simulink model "03_ee_c"  (R2023a)
settings: Solver=VariableStepDiscrete  StartTime=0.0  StopTime=6  RelTol=1e-4
PreLoadFcn:
  | Ts=10e-6;
  | fnom=50;
undefined symbols (not defined in the file): D1, D11, Delta, DiscIntNeverNeededParam, find_system
libraries: powerlib_extras x18, simulink_extras x7, spsThreePhaseVIMeasurementLib x6, spsThreePhaseTransformerTwoWindingsLib x2, spsUniversalBridgeLib x2, spsThreePhaseProgrammableVoltageSourceLib x1, spsThreePhaseMutualInductanceZ1Z0Lib x1, spsThreePhasePISectionLineLib x1, spsGroundLib x1, spsSeriesRLCBranchLib x1, spsThreePhaseSeriesRLCBranchLib x1, spsThreePhaseSeriesRLCLoadLib x1
(part 1 of 3)
Description:
  | Copyright 2008-2009 The MathWorks(TM), Inc.
settings Model: SimulationMode=accelerator  Creator=ch0272  LastModifiedBy=eagle
settings SolverCC: AlgebraicLoopSolver=TrustRegion  SolverResetMethod=Robust
settings DataIOCC: LimitDataPoints=on  SaveFinalState=on  SaveFormat=StructureWithTime  SignalLoggingSaveFormat=ModelDataLogs  ReturnWorkspaceOutputs=off
settings OptimizationCC: ExpressionDepthLimit=2147483647  InitFltsAndDblsToZero=on  LifeSpan=inf
settings DebuggingCC: UnderspecifiedInitializationDetection=Classic  MergeDetectMultiDrivingBlocksExec=none  SolverPrmCheckMsg=warning  FcnCallInpInsideContextMsg=warning  StateNameClashWarn=warning  SFUnexpectedBacktrackingDiag=warning  SFNoUnconditionalDefaultTransitionDiag=warning  SFExecutionAtInitializationDiag=none  ArithmeticOperatorsInVariantConditions=warning
settings HardwareCC: ProdBitPerPointer=32  ProdBitPerSizeT=32  ProdBitPerPtrDiffT=32  ProdLargestAtomicFloat=None  ProdIntDivRoundTo=Undefined  ProdEndianess=Unspecified  ProdWordSize=32  ProdHWDeviceType=32-bit Generic
settings ModelReferenceCC: PropagateSignalLabelsOutOfModel=off
settings SFSimCC: SimUseLocalCustomCode=off  CustomCodeUndefinedFunction=UseInterfaceOnly
settings RTWCC: RTWUseLocalCustomCode=off
settings CodeAppCC: StateflowObjectComments=on
settings GRTTargetCC: TargetLangStandard=C89/C90 (ANSI)  CombineOutputUpdateFcns=off  GRTInterface=on
settings ConfigComp: CovMetricSettings=dw  CovSaveCumulativeToWorkspaceVar=on  CovSaveSingleToWorkspaceVar=on  CovExternalEMLEnable=off  CovSFcnEnable=off
settings SimscapeCC: SimscapeNormalizeSystem=off

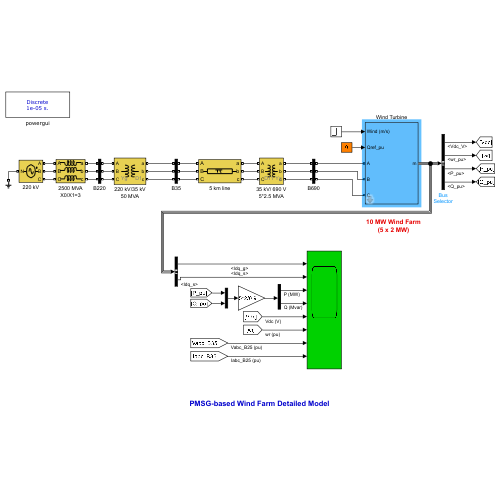
[thumbnail: Simulink's stored preview of the top-level diagram]
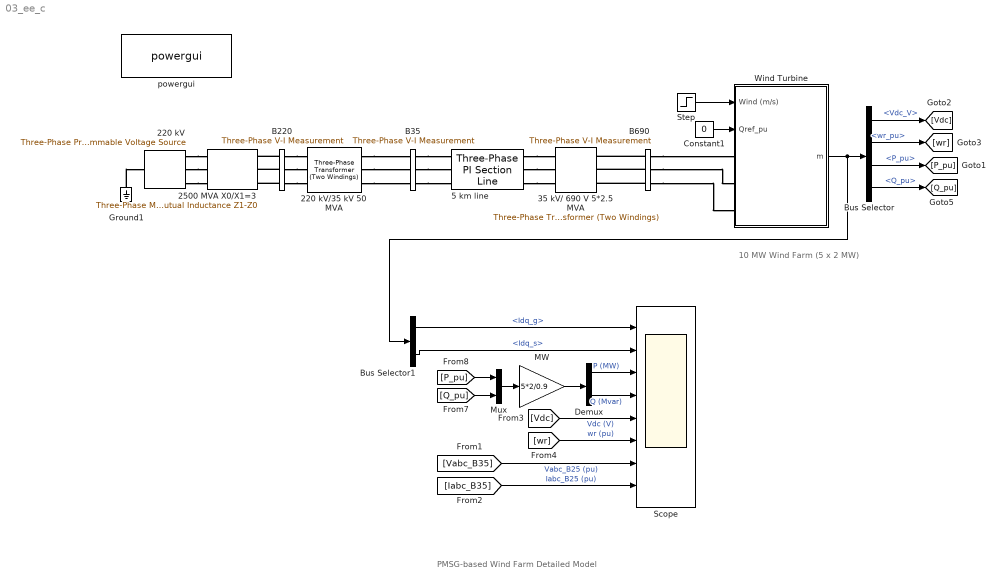
== system 03_ee_c ==
  note: 10 MW Wind Farm
      | (5 x 2 MW)
  note: PMSG-based Wind Farm Detailed Model
  220 kV : spsThreePhaseProgrammableVoltageSourceLib/Three-Phase Programmable Voltage Source  PositiveSequence=[220e3 0 fnom]  VariationEntity=Amplitude  VariationType=Table of time-amplitude pairs  VariationTypeAlt=Step  VariationStep=-0.2  VariationRate=10  VariationMagnitude=0.3  VariationFrequency=2  VariationTiming=[0.05 0.05+5/60]  VariationPhaseA=off  Amplitudes=[1 0.4 1.0]  TimeValues=[0 4 4.625]  HarmonicGeneration=off  HarmonicA=[1 -0.1 0 2]  HarmonicB=[2 0.15 35 2]*0  Timing="[0.1  2]"  BusType=swing  Pref=0  Qref=0  Qmin=-inf  Qmax=inf
  220 kV/35 kV 50 MVA : spsThreePhaseTransformerTwoWindingsLib/Three-Phase Transformer (Two Windings)  Winding1Connection=Yg  Winding2Connection=Delta (D1)  CoreType=Three single-phase transformers  SetSaturation=off  Hysteresis=off  DataFile='basic_model'  SetInitialFlux=off  Measurements=None  UNITS=pu  NominalPower=[50e6 fnom ]  Winding1="[ 220e3  0.08/30   0.05 ]"  Winding2="[ 35e3  0.08/30  0.05]"  Rm=500  Lm=500  L0=0.5  Saturation="[ 0,0  ;  0.005,1.2  ;  1.0,1.4 ]"  InitialFluxes=[ 0.8 , -0.8 , 0.7 ]  BreakLoop=off  DiscreteSolver=Trapezoidal iterative  DataType=off  TransfoNumber=0
  2500 MVA X0/X1=3 : spsThreePhaseMutualInductanceZ1Z0Lib/Three-Phase Mutual Inductance Z1-Z0  LConnTagsString=a|b|c  RConnTagsString=A|B|C  PositiveSequence="[0.1  1.0/(2*pi*fnom)] *220e3^2/2500e6"  ZeroSequence="[0.3  3.0/(2*pi*fnom)] *220e3^2/2500e6"
      settings: AttributesFormatString=\n
      settings: LibrarySourceBlock=|
      | sps_lib/Power Grid Elements/Three-Phase
      | Mutual Inductance
      | Z1-Z0
  35 kV/ 690 V 5*2.5 MVA : spsThreePhaseTransformerTwoWindingsLib/Three-Phase Transformer (Two Windings)  Winding1Connection=Delta (D11)  Winding2Connection=Yg  CoreType=Three single-phase transformers  SetSaturation=off  Hysteresis=off  DataFile='hysteresis'  SetInitialFlux=off  Measurements=None  UNITS=pu  NominalPower="[2.5e6*5  fnom]"  Winding1=[35e3 , 0.025/30 , 0.025]  Winding2=[ 690, 0.025/30 , 0.025]  Rm=500  Lm=inf  L0=0.5  Saturation=[ 0,0 ; 0.0024,1.2 ; 1.0,1.52 ]  InitialFluxes=[ 0.8 , -0.8 , 0.7 ]  BreakLoop=off  DiscreteSolver=Trapezoidal iterative  DataType=off  TransfoNumber=0
  5 km line : spsThreePhasePISectionLineLib/Three-Phase PI Section Line  LConnTagsString=a|b|c  RConnTagsString=A|B|C  Length=5  Frequency=50  Resistances=[0.1153 0.413]  Inductances=[1.05e-3 3.32e-3]  Capacitances=[11.33e-009 5.01e-009]
  B220 : spsThreePhaseVIMeasurementLib/Three-Phase V-I Measurement  VoltageMeasurement=no  SetLabelV=off  LabelV=Vabc_B120  Vpu=off  VpuLL=off  CurrentMeasurement=no  SetLabelI=on  LabelI=Iabc_B120  Ipu=off  Pbase=100e6  Vbase=120e3  OutputType=Complex  PhasorSimulation=off  PSBequivalent=0
  B35 : spsThreePhaseVIMeasurementLib/Three-Phase V-I Measurement  VoltageMeasurement=phase-to-ground  SetLabelV=on  LabelV=Vabc_B35  Vpu=on  VpuLL=off  CurrentMeasurement=yes  SetLabelI=on  LabelI=Iabc_B35  Ipu=on  Pbase=10e6  Vbase=35e3  OutputType=Complex  PhasorSimulation=off  PSBequivalent=0
  B690 : spsThreePhaseVIMeasurementLib/Three-Phase V-I Measurement  VoltageMeasurement=phase-to-ground  SetLabelV=on  LabelV=Vabc_B690  Vpu=on  VpuLL=off  CurrentMeasurement=yes  SetLabelI=on  LabelI=Iabc_B690  Ipu=on  Pbase=5*2e6  Vbase=690  OutputType=Complex  PhasorSimulation=off  PSBequivalent=0
  Bus Selector : BusSelector  OutputSignals=Vdc_V,Stator dq Frame.wr_pu,PQ&V.P_pu,PQ&V.Q_pu
  Bus Selector1 : BusSelector  OutputSignals=Grid dq Frame.Idq_g,Stator dq Frame.Idq_s
  Constant1 : Constant  Value=0
  Demux : Demux  Outputs=2
  Ground1 : spsGroundLib/Ground  LConnTagsString=a
  MW : Gain  Gain=5*2/0.9  SaturateOnIntegerOverflow=on  OutDataTypeStr=Inherit: Same as input  ParamDataTypeStr=Inherit: Same as input
  Mux : Mux  Inputs=2
  Scope : Scope  NumInputPorts=8
  Step : Step  Time=3  Before=11  After=11  SampleTime=0
  Wind Turbine : Subsystem  AncestorBlock=|  LoadFcn=%find_system(gcs,'FollowLinks', 'on', 'LookUnderMasks', 'all');  mask(Wind Turbine: Model 7){Nb_wt=5, ShowParameters=Turbine data for 1 wind turbine, nom=[2e6/0.9 690 fnom], Reactances=[ 0.0014 0.0014 ], Rs=0.0066, Flux=8.5, mec=[5e4 0 38], Vnom=690, Imax_grid_conv=1.1, RL_grid=[ 0.15 0.15/50], C_var_filter1=150e3, Vdc_nom=1200, C_DClink1=50000e-6, L_R_Boost=[0.0012     5e-3], Pmec1=2e6, wind_speed_CpMax=11, wind0=11, DisplayTurbChar=off, H_WT=4.32, Ksh=0.3, D_mutual=1.5, w_wt0=1, torque0=1, Kdc=[1.1   27.5], Ki_var_reg=0.05, Ki_volt_reg=2, Kgrid_side_cur_reg=[2  50], Kspeed=[5 20], K_PMSG_cur_reg=[2 50], Kp_pitch=15, Kcompensation=[1.5  6], pitch_max=27, pitch_rate=10, Ts=Ts}
      | DRlib/Wind Generation/Wind Turbine
      | Induction Generator
      | (Phasor Type)
      mask prompts: Nb_wt "Number of wind turbines:"; ShowParameters "Display:"; nom "Nom. power, L-L volt. and freq.: [Pn (VA), Vn (Vrms), fn (Hz)]"; Reactances "Reactances [Ld Lq] (p.u.):"; Rs "Resistance Rs :"; Flux "Flux linkage estableished by magnets"; mec "Inertia constant, friction factor, and pairs of poles: [ J  F  p ]"; Vnom "Grid-side converter nominal AC voltage (V):"; Imax_grid_conv "Grid-side converter maximum AC current (pu based on generator power and converter nominal AC voltage):"; RL_grid "Grid-side coupling inductor [ L(pu) R(pu),pu based on generator power and converter nominal AC voltage] :"; C_var_filter1 "Line filter capacitor (Q=50) (var):"; Vdc_nom "Nominal DC bus voltage (V)"; C_DClink1 "DC bus capacitor (F):"; L_R_Boost "Boost converter inductance [L(H) R(ohm)]:"; Pmec1 "Nominal mechanical output power (W):"; wind_speed_CpMax "Wind speed at nominal speed and at Cp max (must be between 6 m/s and 30 m/s) (m/s):"; wind0 "Initial wind speed (m/s):"; DisplayTurbChar "Display wind turbine power characteristics:"; H_WT "Wind turbine inertia constant H (s):"; Ksh "Shaft spring constant refer to high-speed shaft (pu of nominal mechanical torque/rad):"; D_mutual "Shaft mutual damping (pu of nominal mechanical torque/pu dw):"; w_wt0 "Turbine initial speed (pu of nominal speed):"; torque0 "Initial output torque (pu of nominal mechanical torque):"; Kdc "DC bus voltage regulator gains [Kp Ki]:"; Ki_var_reg "Grid-side converter var regulator gain [ Ki]:"; Ki_volt_reg "Grid-side converter voltage regulator gain [ Ki]:"; Kgrid_side_cur_reg "Grid-side converter current regulator gains [Kp Ki]:"; Kspeed "Speed regulator gains [Kp Ki]:"; K_PMSG_cur_reg "Stator-side converter current regulator gains [Kp Ki]:"; Kp_pitch "Pitch controller gain [Kp]:"; Kcompensation "Pitch compensation gains [Kp Ki]:"; pitch_max "Maximum pitch angle (deg):"; pitch_rate "Maximum rate of change of pitch angle (deg/s)"; Ts "Sample time (s):"
      mask help: This block implements a model of a variable speed pitch controlled wind turbine using a synchronous generator.
      mask init:
      | %Generator data
      | Pnom=nom(1)*Nb_wt;
      | Vnom_gen=nom(2);
      | Fnom=nom(3);
      | Ld=Reactances(1)/Nb_wt;
      | Lq=Reactances(2)/Nb_wt;
      | Resistance=Rs/Nb_wt;
      | J=mec(1)*Nb_wt;
      | F=mec(2);
      | p=mec(3);
      | 
      | % Converters data
      | L_RL=RL_grid(1);
      | R_RL=RL_grid(2);
      | L_Boost=L_R_Boost(1)/Nb_wt;
      | R_Boost=L_R_Boost(2)/Nb_wt;
      | Q_filter=50;
      | C_DClink=C_DClink1*Nb_wt;
      | C_var_filter=C_var_filter1*Nb_wt;
      | 
      | % Controller data
      | Freq_filter=10000;   %Hz
      | Zeta_filter=0.707;
      | Kp_dc=Kdc(1);
      | Ki_dc=Kdc(2);
      | Kp_grid_side_cur_reg=Kgrid_side_cur_reg(1);
      | Ki_grid_side_cur_reg=Kgrid_side_cur_reg(2);
      | Kp_speed=Kspeed(1);
      | Ki_speed=Kspeed(2);
      | Kp_PMSG_side_cur_reg=K_PMSG_cur_reg(1);
      | Ki_PMSG_side_cur_reg=K_PMSG_cur_reg(2);
      | Kp_compensation=Kcompensation(1);
      | Ki_compensation=Kcompensation(2);
      | Mod_index_max=1.1;
      | T_speed=5;      %Speed reference time constant (s)
      | Iq_ref_limit_time_constant=0.3; %(s)
      | Current_reg_output_limit=1.1;   %(pu)
      | Var_reg_output_hi_limit=1.1;    %(pu)
      | Var_reg_output_low_limit=0.9;   %(pu)
      | Pitch_time_constant=0.01;       %(s)
      | Freq_PWM=3000; %Hz, Inverter
      | Ts_snub=50e-6;  %Sample time to compute snubber resistance
      | 
      | 
      | % Turbine data
      | Pmec=Pmec1*Nb_wt;
      | c1 = 0.6450;
      | c2 = 116;
      | c3 = .4;
      | c4 = 5;
      | c5 = 21;
      | c6 = .00912;  % Set Pmin in stall condition (does not vary with wind_speed_Pmax)
      | c7 = .08;
      | c8 = .035;
      | theta=0;
      | CpMax=.5;
      | lambda_CpMax=9.9495;
      | 
      | c1_c8=[c1 c2 c3 c4 c5 c6 c7 c8];
      |   
      | 
      | %   Cp = c1*(c6*lambda + (-c4 - c3*(2.5 + theta) + c2*(1/(lambda + ...
      | %   c7*(2.5 + theta)) - c8/(1 + (2.5 + theta)^3)))/exp(c5*(1/(lambda + ...
      | %   c7*(2.5 + theta)) - c8/(1 + (2.5 + theta)^3))))
      | 
      | 
      |         %%%%%%%%%%%%%%%%%%%%%%%%%%%%%%%%%%%%%%%%%%%%%%%%%%%%%%%%%%%%%%%%%%%%%%%%%%%
      |         % Operation at Cp max
      |         %%%%%%%%%%%%%%%%%%%%%%%%%%%%%%%%%%%%%%%%%%%%%%%%%%%%%%%%%%%%%%%%%%%%%%%%%%%
      |         
      |         rated_omegar=1;
      |         omegar = rated_omegar;
      |         
      |         % Enforce boundaries on wind speed
      |         % A warning could be displayed
      |         if wind_speed_CpMax < 6
      |             wind_speed_CpMax=6;
      |             disp('Warning: Wind speed at nominal speed and at Cp max has been set to 6 m/s')
      |         end
      |         if wind_speed_CpMax > 30
      |             wind_speed_CpMax=30;
      |             disp('Warning: Wind speed at nominal speed and at Cp max has been set to 30 m/s')
      |         end
      | 
      |         K1=lambda_CpMax/omegar*wind_speed_CpMax;
      |         
      |         % Calculation of K2 needed to get P equal to the requested value at
      |         % Cp max for the requested wind speed
      |         
      |         Prated=Pmec;
      |         P_rated_omegar_theta_zero=0.75;
      |         
      |         K2 = P_rated_omegar_theta_zero*Prated/(wind_speed_CpMax^3*CpMax);
      |         
      |         K1_K2=[K1 K2];
      |         
      |         %%%%%%%%%%%%%%%%%%%%%%%%%%%%%%%%%%%%%%%%%%%%%%%%%%%%%%%%%%%%%%%%%%%%%%%%%%%
      |         % End of calculation for operation at Cp max
      |         %%%%%%%%%%%%%%%%%%%%%%%%%%%%%%%%%%%%%%%%%%%%%%%%%%%%%%%%%%%%%%%%%%%%%%%%%%%
      |         
      | 
      | %%%%%%%%%%%%%%%%%%%%%%%%%%%%%%%%%%%%%%%%%%%%%%%%%%%%%%%%%%%%%%%%%%%%%%%%%%%
      | % Plot turbine characteristics
      | %%%%%%%%%%%%%%%%%%%%%%%%%%%%%%%%%%%%%%%%%%%%%%%%%%%%%%%%%%%%%%%%%%%%%%%%%%% 
      | 
      | DisplayTurbChar=get_param(gcb,'DisplayTurbChar');
      | if strcmp(DisplayTurbChar,'on')
      |     vect_theta = 0:2:30;
      |     
      |     vect_lambda = 1:0.2:30;
      |     
      |     clear Cp;
      |     
      |     for i=1:length(vect_theta)
      |      for j=1:length(vect_lambda)
      |                 Cp(i,j) = c1*(c6*vect_lambda(j) + (-c4 - c3*(2.5 + vect_theta(i)) + c2*(1/(vect_lambda(j) + ...
      |                 c7*(2.5 + vect_theta(i))) - c8/(1 + (2.5 + vect_theta(i))^3)))/exp(c5*(1/(vect_lambda(j) + ...
      |                 c7*(2.5 + vect_theta(i))) - c8/(1 + (2.5 + vect_theta(i))^3))));
      |      end
      |     end
      | 
      |     figure(1);
      |     clf;
      |     hold on;
      | 
      |     plot(vect_lambda, Cp);
      |     axis([0, 25, 0, .6]);
      |     title('Wind Turbine Cp Characteristic (pitch angle increases by step of 2 deg.)');
      |     ylabel('Cp');
      |     set(gca,'ytick',[0 .1 .2 .3 .4 .5 .6]);
      |     xlabel('Lambda');
      |     grid on;
      |     text(10.1,0.51,'Pitch angle 0 degree');
      | 
      |     hold off
      |     
      |     % Plot of the wind turbine mechanical power output (pu) lambda and Cp
      |     % characteristics against wind speed (m/s) for a range of theta.
      |     
      |     wind_speed_range = [1,.2,30];
      |     vect_wind_speed = 1:0.2:30;
      |     
      |     clear lambda;
      |     clear Cp;
      |     clear P;
      | 
      |     for i=1:length(vect_theta)
      |         for j=1:length(vect_wind_speed)
      |             lambda(i,j) = K1*omegar/vect_wind_speed(j);
      |             Cp(i,j) = c1*(c6*lambda(i,j) + (-c4 - c3*(2.5 + vect_theta(i)) + c2*(1/(lambda(i,j) + ...
      |             c7*(2.5 + vect_theta(i))) - c8/(1 + (2.5 + vect_theta(i))^3)))/exp(c5*(1/(lambda(i,j) + ...
      |             c7*(2.5 + vect_theta(i))) - c8/(1 + (2.5 + vect_theta(i))^3))));
      |             P(i,j) = K2/Prated*vect_wind_speed(j)^3*Cp(i,j);
      |         end
      |     end
      |     
      |     
      |     figure(2);
      |     clf;
      |     hold on
      |     
      |     subplot(3,1,1);
      |     plot(vect_wind_speed, P);
      |     axis([0, 35, 0, 1.5]);
      |     title('Wind Turbine Characteristics (w = 1 pu, pitch angle increases by step of 2 deg.)');
      |     ylabel('P (pu)');
      |     set(gca,'ytick',0:.5:4);
      |     grid on;
      |     
      |     subplot(3,1,2);
      |     plot(vect_wind_speed, lambda);
      |     axis([0, 35, 0, 20]);
      |     ylabel('Lambda');
      |     grid on;
      |     
      |     subplot(3,1,3)
      |     plot(vect_wind_speed, Cp);
      |     axis([0, 35, 0, .6]);
      |     xlabel('Wind Speed (m/s)');
      |     ylabel('Cp');
      |     set(gca,'ytick',[0 .1 .2 .3 .4 .5 .6]);
      |     grid on;
      | 
      |     hold off
      |     set_param(gcb,'DisplayTurbChar','off')
      |     
      | end
      mask TypeOptions ShowParameters: Generator data for 1 wind turbine | Converters data for 1 wind turbine | Turbine data for 1 wind turbine | Drive train data for 1 wind turbine | Control parameters for 1 wind turbine
      mask Callback ShowParameters:
      | BlockName=getfullname(gcb);
      | %
      | Param_Show=get_param(BlockName,'ShowParameters');
      | Param_DisplayTurbChar=get_param(BlockName,'DisplayTurbChar');
      | 
      | p_mask{3}='off';p_mask{4}='off';p_mask{5}='off';
      | p_mask{6}='off';p_mask{7}='off';p_mask{8}='off';p_mask{9}='off';
      | p_mask{10}='off';p_mask{11}='off';p_mask{12}='off';p_mask{13}='off';
      | p_mask{14}='off';p_mask{15}='off';p_mask{16}='off';p_mask{17}='off';
      | p_mask{18}='off';p_mask{19}='off';p_mask{20}='off';p_mask{21}='off';
      | p_mask{22}='off';p_mask{23}='off';p_mask{24}='off';p_mask{25}='off';
      | p_mask{26}='off';p_mask{27}='off';p_mask{28}='off';p_mask{29}='off';
      | p_mask{30}='off';p_mask{31}='off';p_mask{32}='off';p_mask{33}='off';
      | 
      | switch Param_Show
      | 	case 'Generator data for 1 wind turbine'
      | 		p_mask{3}='on';p_mask{4}='on';p_mask{5}='on';
      |         p_mask{6}='on';p_mask{7}='on';
      |     case 'Converters data for 1 wind turbine'
      | 		p_mask{8}='on';p_mask{9}='on';
      |         p_mask{10}='on';p_mask{11}='on';
      |         p_mask{12}='on';p_mask{13}='on';p_mask{14}='on';
      | 	case 'Turbine data for 1 wind turbine'
      | 		p_mask{15}='on';p_mask{16}='on';
      |         p_mask{17}='on';p_mask{18}='on';
      |     case 'Drive train data for 1 wind turbine'
      |         p_mask{19}='on';p_mask{20}='on';
      |         p_mask{21}='on';p_mask{22}='on';p_mask{23}='on';
      |     case 'Control parameters for 1 wind turbine'
      |         p_mask{24}='on';p_mask{25}='on';p_mask{26}='on';p_mask{27}='on';
      |         p_mask{28}='on';p_mask{29}='on';p_mask{30}='on';p_mask{31}='on';
      |         p_mask{32}='on';p_mask{33}='on';
      | end
      | 
      | ParVisible={'on','on',p_mask{3},p_mask{4},p_mask{5},p_mask{6},...
      |     p_mask{7},p_mask{8},p_mask{9},p_mask{10},p_mask{11},p_mask{12},...
      |     p_mask{13},p_mask{14},p_mask{15},p_mask{16},p_mask{17},p_mask{18},...
      |     p_mask{19},p_mask{20},p_mask{21},p_mask{22},p_mask{23},p_mask{24},...
      |     p_mask{25},p_mask{26},p_mask{27},p_mask{28},p_mask{29},p_mask{30},...
      |     p_mask{31},p_mask{32},p_mask{33},'on'};
      | %
      | set_param(BlockName,'MaskVisibilities',ParVisible);
      | set_param(BlockName,'DisplayTurbChar',Param_DisplayTurbChar);
      mask Display: disp(' ');
  powergui : sps_lib/powergui  SimulationMode=Discrete  SampleTime=Ts  frequency=60  Iterations=50  frequencyindice=50  Pbase=100e6  ErrMax=1e-4  UnitsV=kV  UnitsW=MW  buscounter=0  FunctionMessages=off  echomessages=off  EnableUseOfTLC=off  CurrentSourceSwitches=off  DisableSnubberDevices=off  DisableRonSwitches=off  DisableVfSwitches=off  DisplayEquations=off  AutomaticDiscreteSolvers=off  SolverType=Tustin  Interpol=off  ExternalGateDelay=off  methode=off  Ts=0  x0status=blocks  SPID=off  SwTol=0  HookPort=off  NonlinearTolerance=1e-4  nMaxIteration=100  ContinueOnMaxIteration=off  RestoreLinks=warning  ResistiveCurrentMeasurement=off  Frange=[0:2:500]  Ylog=off  Xlog=on  ShowGrid=off  save=off  variable=ZData  structure=0  ZoomFFT=on  StartTime=0.0  cycles=1  DisplayStyle=1  fundamental=60  FreqAxis=off  MaxFrequency=1000  frequencyindicesteady=1  RmsSteady=1  display=off
  wires:
  Step/1 -> Wind Turbine/1("Wind (m/s) ")
  Wind Turbine/1(m) -> Bus Selector1/1, Bus Selector/1
  Constant1/1 -> Wind Turbine/2(Qref_pu)
  Bus Selector1/1 -> Scope/1  "<Idq_g>"
  Demux/1 -> Scope/3  "P (MW)"
  Demux/2 -> Scope/4  "Q (Mvar)"
  [Vdc] -> Scope/5  "Vdc (V)"
  [wr] -> Scope/6  "wr (pu)"
  [Vabc_B35] -> Scope/7  "Vabc_B25 (pu)"
  [Iabc_B35] -> Scope/8  "Iabc_B25 (pu)"
  [Q_pu] -> Mux/2
  [P_pu] -> Mux/1
  Mux/1 -> MW/1
  MW/1 -> Demux/1
  Bus Selector/1 -> [Vdc]  "<Vdc_V>"
  Bus Selector/2 -> [wr]  "<wr_pu>"
  Bus Selector/3 -> [P_pu]  "<P_pu>"
  Bus Selector/4 -> [Q_pu]  "<Q_pu>"
  Bus Selector1/2 -> Scope/2  "<Idq_s>"
  connections:
  220 kV/35 kV 50 MVA/RConn2 -- B35/LConn2
  220 kV/35 kV 50 MVA/RConn3 -- B35/LConn3
  220 kV/35 kV 50 MVA/RConn1 -- B35/LConn1
  B690/LConn2 -- 35 kV/ 690 V 5*2.5 MVA/RConn2
  B690/LConn1 -- 35 kV/ 690 V 5*2.5 MVA/RConn1
  B690/LConn3 -- 35 kV/ 690 V 5*2.5 MVA/RConn3
  220 kV/RConn1 -- 2500 MVA X0/X1=3/LConn1
  220 kV/RConn2 -- 2500 MVA X0/X1=3/LConn2
  220 kV/RConn3 -- 2500 MVA X0/X1=3/LConn3
  B220/LConn1 -- 2500 MVA X0/X1=3/RConn1
  B220/LConn2 -- 2500 MVA X0/X1=3/RConn2
  B220/LConn3 -- 2500 MVA X0/X1=3/RConn3
  B220/RConn1 -- 220 kV/35 kV 50 MVA/LConn1
  B220/RConn2 -- 220 kV/35 kV 50 MVA/LConn2
  B220/RConn3 -- 220 kV/35 kV 50 MVA/LConn3
  B35/RConn1 -- 5 km line/LConn1
  B35/RConn2 -- 5 km line/LConn2
  B35/RConn3 -- 5 km line/LConn3
  5 km line/RConn1 -- 35 kV/ 690 V 5*2.5 MVA/LConn1
  5 km line/RConn2 -- 35 kV/ 690 V 5*2.5 MVA/LConn2
  5 km line/RConn3 -- 35 kV/ 690 V 5*2.5 MVA/LConn3
  B690/RConn1 -- Wind Turbine/LConn1
  B690/RConn2 -- Wind Turbine/LConn2
  B690/RConn3 -- Wind Turbine/LConn3
  Ground1/LConn1 -- 220 kV/LConn1

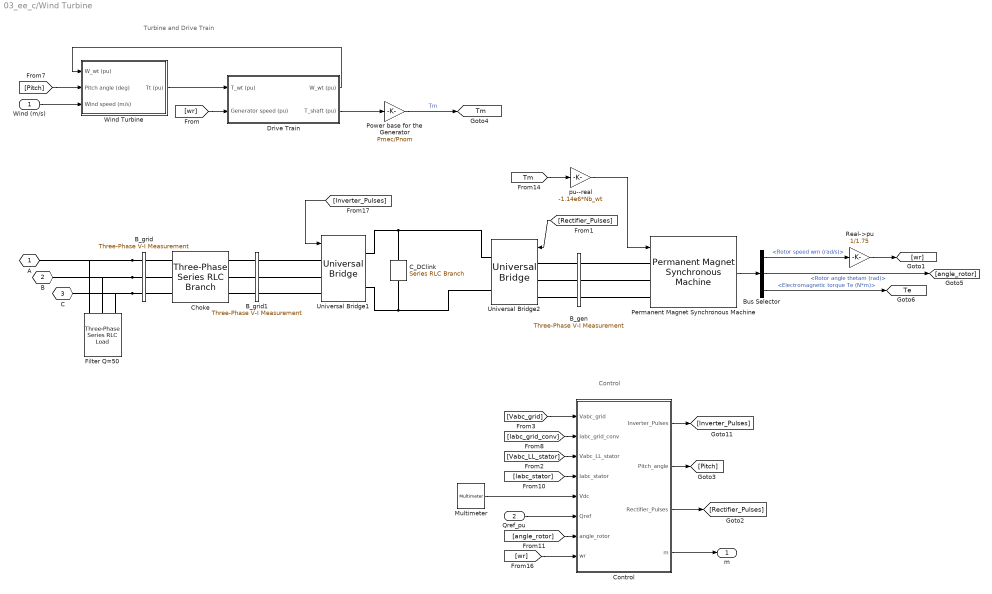
== system 03_ee_c/Wind Turbine ==
  note: Turbine and Drive Train
  note: Control
  "Wind (m/s) " : Inport
  Qref_pu : Inport  Port=2
  B_gen : spsThreePhaseVIMeasurementLib/Three-Phase V-I Measurement  VoltageMeasurement=phase-to-phase  SetLabelV=on  LabelV=Vabc_LL_stator  Vpu=on  VpuLL=off  CurrentMeasurement=yes  SetLabelI=on  LabelI=Iabc_stator  Ipu=on  Pbase=Pnom  Vbase=Vnom_gen  OutputType=Complex  PhasorSimulation=off  PSBequivalent=0
  B_grid : spsThreePhaseVIMeasurementLib/Three-Phase V-I Measurement  VoltageMeasurement=phase-to-ground  SetLabelV=on  LabelV=Vabc_grid  Vpu=on  VpuLL=off  CurrentMeasurement=yes  SetLabelI=on  LabelI=Iabc_grid_conv  Ipu=on  Pbase=Pnom  Vbase=Vnom  OutputType=Complex  PhasorSimulation=off  PSBequivalent=0
  B_grid1 : spsThreePhaseVIMeasurementLib/Three-Phase V-I Measurement  VoltageMeasurement=phase-to-ground  SetLabelV=on  LabelV=Vabc_grid_conv  Vpu=on  VpuLL=off  CurrentMeasurement=no  SetLabelI=on  LabelI=Iabc_grid_conv  Ipu=on  Pbase=Pnom  Vbase=Vnom  OutputType=Complex  PhasorSimulation=off  PSBequivalent=0
  Bus Selector : BusSelector  OutputSignals=Rotor speed wm (rad/s),Rotor angle thetam (rad),Electromagnetic torque Te (N*m)
  C_DClink : spsSeriesRLCBranchLib/Series RLC Branch  LConnTagsString=__new0  RConnTagsString=__new0  BranchType=C  Resistance=1  Inductance=1e-3  SetiL0=off  InitialCurrent=0  Capacitance=C_DClink  Setx0=on  InitialVoltage=Vdc_nom  Measurements=Branch voltage
  "Choke " : spsThreePhaseSeriesRLCBranchLib/Three-Phase Series RLC Branch  LConnTagsString=A|B|C  RConnTagsString=A|B|C  BranchType=RL  Resistance=R_RL*Vnom^2/Pnom  Inductance=L_RL*Vnom^2/Pnom/(2*pi*Fnom)  Capacitance=[]  Measurements=None
  Control : Subsystem
  Drive Train : Subsystem  mask(Wind Turbine shaft){H_WT=H_WT, Ksh=Ksh, D_mutual=D_mutual, wbase=2*pi*Fnom/p, w_wt0=w_wt0, torque0=torque0, Ts=Ts}
      mask prompts: H_WT "Wind turbine inertia constant H (s):"; Ksh "Shaft spring constant (pu of nominal mechanical torque/rad):"; D_mutual "Shaft mutual damping (pu of nominal mechanical torque/pu dw):"; wbase "Shaft base speed (rad/s):"; w_wt0 "Turbine initial speed (pu of base speed):"; torque0 "Initial output torque (pu of nominal mechanical torque):"; Ts "Sample time (s):"
      mask help:
      | This block implements a wind turbine drive train model. All shaft parameters are referred to high-speed shaft (generator shaft).
      |
      | The first input is the wind turbine torque in per unit (pu) based on the nominal power of the turbine and the base speed of the generator. The second input is the generator speed in pu based on the base speed of the generator.
      |
      | The outputs are:
      | 1- the transmitted torque of the shaft in pu based on the nominal power of the turbine and the base speed of the generator.
      | 2- the wind turbine speed in pu of the base speed of the generator.
  Filter Q=50 : spsThreePhaseSeriesRLCLoadLib/Three-Phase Series RLC Load  LConnTagsString=A|B|C  Configuration=Y (grounded)  NominalVoltage=Vnom  Vabc=[1e3 1e3 1e3]  Vabcp=[1e3 1e3 1e3]  NominalFrequency=Fnom  UnbalancedPower=off  ActivePower=C_var_filter/Q_filter  InductivePower=0  CapacitivePower=C_var_filter  Pabc=[10e3 9e3 11e3]  QLabc=[100 90 110]  QCabc=[100 90 110]  Pabcp=[10e3 9e3 11e3]  QLabcp=[100 90 110]  QCabcp=[100 90 110]  Measurements=None  LoadType=constant Z
  Multimeter : spsMultimeterLib/Multimeter  L=1  sel=1  yselected={}  Gain=1  OutputType=Complex  PlotAtSimulationStop=off  PhasorSimulation=off
  Permanent Magnet Synchronous Machine : spsPermanentMagnetSynchronousMachineLib/Permanent Magnet Synchronous Machine  NbPhases=3  FluxDistribution=Sinusoidal  RotorType=Salient-pole  MechanicalLoad=Torque Tm  PresetModel=No  ShowDetailedParameters=on  MeasurementBus=off  Resistance=Resistance  Inductance=8.5e-3  dqInductances=[Ld Lq]  La=0.000835  MachineConstant=Flux linkage established by magnets (V.s)  Flux=8.85  VoltageCst=60998.0726  TorqueCst=504.45  Flat=120  Mechanical=[J F p]  PolePairs=38  InitialConditions=[1.75,0, 0,0]  InitialConditions5ph=[0 0 0 0 0 0]  RefAngle=90 degrees behind phase A axis (modified Park)  IterativeDiscreteModel=Trapezoidal non iterative  TsBlock=-1  TsPowergui=0
  Power base for the Generator : Gain  Gain=Pmec/Pnom  SaturateOnIntegerOverflow=on  OutDataTypeStr=Inherit: Same as input  ParamDataTypeStr=Inherit: Same as input
  Real->pu : Gain  Gain=1/1.75  SaturateOnIntegerOverflow=on  OutDataTypeStr=Inherit: Same as input  ParamDataTypeStr=Inherit: Same as input
  Universal Bridge1 : spsUniversalBridgeLib/Universal Bridge  Arms=3  SnubberResistance=1e6/Nb_wt  SnubberCapacitance=inf  Device=IGBT / Diodes  Ron=1e-6/Nb_wt  Lon=0  ForwardVoltages="[  0  0  ]"  ForwardVoltage=0  GTOparameters=[ 10e-6 , 20e-6 ]  IGBTparameters=[ 1e-6 , 2e-6 ]*0  Measurements=None  Measurements_2=None  converterType=Rectifier
  Universal Bridge2 : spsUniversalBridgeLib/Universal Bridge  Arms=3  SnubberResistance=1e6/Nb_wt  SnubberCapacitance=inf  Device=IGBT / Diodes  Ron=1e-6/Nb_wt  Lon=0  ForwardVoltages="[  0  0  ]"  ForwardVoltage=0  GTOparameters=[ 10e-6 , 20e-6 ]  IGBTparameters=[ 1e-6 , 2e-6 ]*0  Measurements=None  Measurements_2=None  converterType=Rectifier
  Wind Turbine : Subsystem  AncestorBlock=DRlib/Wind Generation/Wind Turbine  mask(Wind Turbine){Prated=Pmec, c1_c8=c1_c8, K1_K2=K1_K2, wind0=wind0, Ts=Ts}
      mask prompts: Prated "Nominal mechanical output power (W):"; c1_c8 "Coefficients [c1 ... c8]"; K1_K2 "Parameters [K1 K2]"; wind0 "Initial wind speed (m/s):"; Ts "Sample time (s):"
      mask help:
      | This block implements a generic wind turbine models.
      |
      | The first input is the turbine speed in per unit of the generator base speed. For a synchronous or asynchronous generator, the base speed is the synchronous speed. For a permanent-magnet generator, the base speed is defined as the speed producing nominal voltage at  no load. The second input is the blade pitch angle in degrees. The third input is the wind speed in m/s.
      |
      | The output is the torque applied to the drive train in per unit based on the nominal power of the turbine and the base speed of the generator.
      mask init:
      | c1 = c1_c8(1);
      | c2 = c1_c8(2);
      | c3 = c1_c8(3);
      | c4 = c1_c8(4);
      | c5 = c1_c8(5);
      | c6 = c1_c8(6);
      | c7 = c1_c8(7);;
      | c8 = c1_c8(8);
      | 
      | K1=K1_K2(1);
      | K2=K1_K2(2);
      settings: OpenFcn=power_openblockproxy();
      mask Display: disp('');
  pu--real : Gain  Gain=-1.14e6*Nb_wt  SaturateOnIntegerOverflow=on  OutDataTypeStr=Inherit: Same as input  ParamDataTypeStr=Inherit: Same as input
  A : PMIOPort  Tag=PMCPort  Side=Left
  B : PMIOPort  Tag=PMCPort  Port=2  Side=Left
  C : PMIOPort  Tag=PMCPort  Port=3  Side=Left
  m : Outport
  tag scope: Te=global, Tm=global
  wires:
  Wind Turbine/1(Tt (pu)) -> Drive Train/1(T_wt (pu))
  [wr] -> Drive Train/2(Generator speed (pu))
  Drive Train/2(T_shaft (pu)) -> Power base for the Generator/1
  Power base for the Generator/1 -> [Tm]  "Tm"
  "Wind (m/s) "/1 -> Wind Turbine/3(Wind speed (m/s))
  Drive Train/1(W_wt (pu)) -> Wind Turbine/1(W_wt (pu))
  [Pitch] -> Wind Turbine/2(Pitch angle (deg))
  Bus Selector/1 -> Real->pu/1  "<Rotor speed wm (rad/s)>"
  [Inverter_Pulses] -> Universal Bridge1/1
  Multimeter/1 -> Control/5(Vdc)
  [Tm] -> pu--real/1
  Permanent Magnet Synchronous Machine/1 -> Bus Selector/1
  Real->pu/1 -> [wr]
  pu--real/1 -> Permanent Magnet Synchronous Machine/1
  [Rectifier_Pulses] -> Universal Bridge2/1
  [Vabc_grid] -> Control/1(Vabc_grid)
  [Iabc_grid_conv] -> Control/2(Iabc_grid_conv)
  [Vabc_LL_stator] -> Control/3(Vabc_LL_stator)
  [Iabc_stator] -> Control/4(Iabc_stator)
  Qref_pu/1 -> Control/6(Qref)
  [angle_rotor] -> Control/7(angle_rotor)
  [wr] -> Control/8(wr)
  Control/1(Inverter_Pulses) -> [Inverter_Pulses]
  Control/2(Pitch_angle) -> [Pitch]
  Control/3(Rectifier_Pulses) -> [Rectifier_Pulses]
  Bus Selector/2 -> [angle_rotor]  "<Rotor angle thetam (rad)>"
  Control/4(m) -> m/1
  Bus Selector/3 -> [Te]  "<Electromagnetic torque Te (N*m)>"
  connections:
  B_grid/RConn1 -- "Choke "/LConn1
  B_grid/RConn2 -- "Choke "/LConn2
  B_grid/RConn3 -- "Choke "/LConn3
  B_grid/LConn1 -- A/RConn1 -- Filter Q=50/LConn1
  B_grid/LConn2 -- Filter Q=50/LConn2 -- B/RConn1
  B_grid/LConn3 -- Filter Q=50/LConn3 -- C/RConn1
  "Choke "/RConn1 -- B_grid1/LConn1
  "Choke "/RConn2 -- B_grid1/LConn2
  "Choke "/RConn3 -- B_grid1/LConn3
  Universal Bridge1/LConn1 -- B_grid1/RConn1
  Universal Bridge1/LConn2 -- B_grid1/RConn2
  Universal Bridge1/LConn3 -- B_grid1/RConn3
  Universal Bridge1/RConn1 -- C_DClink/LConn1 -- Universal Bridge2/RConn1
  Universal Bridge1/RConn2 -- C_DClink/RConn1 -- Universal Bridge2/RConn2
  Permanent Magnet Synchronous Machine/LConn1 -- B_gen/RConn1
  Permanent Magnet Synchronous Machine/LConn2 -- B_gen/RConn2
  Permanent Magnet Synchronous Machine/LConn3 -- B_gen/RConn3
  Universal Bridge2/LConn1 -- B_gen/LConn1
  Universal Bridge2/LConn2 -- B_gen/LConn2
  Universal Bridge2/LConn3 -- B_gen/LConn3

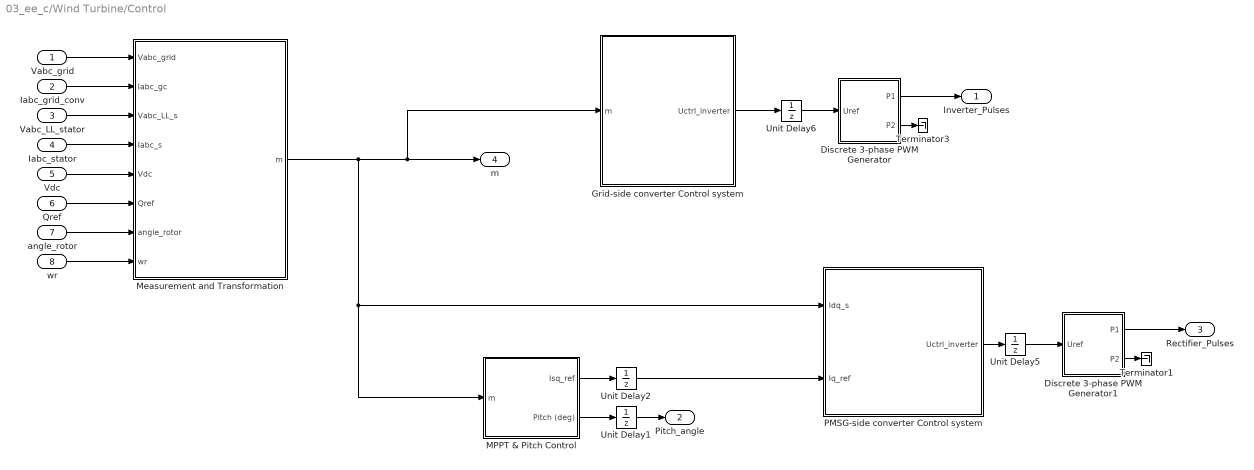
== system 03_ee_c/Wind Turbine/Control ==
  Vabc_grid : Inport
  Iabc_grid_conv : Inport  Port=2
  Vabc_LL_stator : Inport  Port=3
  Iabc_stator : Inport  Port=4
  Vdc : Inport  Port=5
  Qref : Inport  Port=6
  angle_rotor : Inport  Port=7
  wr : Inport  Port=8
  Discrete 3-phase PWM Generator : Subsystem  DialogController=POWERSYS.PowerSysDialog  mask(Discrete 3-phase PWM Generator (2- or 3-level)){ModulatorType=2-level, ModulatorMode=Un-synchronized, nF=27, Fc=Freq_PWM, ModulatingSignals=off, m=0.2, Freq=60, Phase=0, Ts=Ts}
      mask prompts: ModulatorType "Type"; ModulatorMode "Mode of operation"; nF "Switching ratio: chopping frequency / output frequency"; Fc "Carrier frequency (Hz):"; ModulatingSignals "Internal generation of modulating signal(s)"; m "Modulation Index:"; Freq "Output voltage frequency (Hz):"; Phase "Output voltage phase (degrees):"; Ts "Sample time:"
      mask help:
      | The Discrete 3-phase PWM Generator block generates pulses for carrier-based
      | Pulse Width Modulation (PWM) converters. The block can be used to fire the
      | forced-commuted devices (FETs, GTOs, or IGBTs) of 2-level or 3-level converters
      | using a single  bridge or two bridges connected in twin configuration. Vectorized
      | outputs P1 and P2 contain  either 6 pulses (2-level) or 12 pulses (3-level).
      |
      | Use output P1 when operating in single-bridge configuration. The modulating
      | signals can be applied at Input 1 (Uref) and the synchronization signal at input 2 (wt).
      | Look under the mask' of the block to get a description of the pulse pattern.
      mask init:
      | powericon('psbcallbacks',gcb,'Discrete 3-phase PWM Generator');
      | if ModulatorType==1
      |     nPulses=6;
      |     SelectorElements=[1:1:12];
      | else
      |     nPulses=12;
      |  SelectorElements=[1:1:24];
      | end
      | if (ModulatingSignals==1 & ModulatorMode==2),
      |       CmdModulatingSignals=2;
      | else
      |       CmdModulatingSignals=1;
      | end
      | power_initmask();
      mask Help: This block is part of a subset of blocks in the Extras library that does not have documentation associated with it, other than the block mask description.
      mask TypeOptions ModulatorType: 2-level | 3-level
      mask TypeOptions ModulatorMode: Synchronized | Un-synchronized
      mask Callback ModulatorMode: powericon('psbcallbacks',gcb,'Discrete 3-phase PWM Generator',2);
      mask Callback ModulatingSignals: powericon('psbcallbacks',gcb,'Discrete 3-phase PWM Generator',5);
  Discrete 3-phase PWM Generator1 : Subsystem  DialogController=POWERSYS.PowerSysDialog  mask(Discrete 3-phase PWM Generator (2- or 3-level)){ModulatorType=2-level, ModulatorMode=Un-synchronized, nF=27, Fc=Freq_PWM, ModulatingSignals=off, m=0.2, Freq=60, Phase=0, Ts=Ts}
      mask prompts: ModulatorType "Type"; ModulatorMode "Mode of operation"; nF "Switching ratio: chopping frequency / output frequency"; Fc "Carrier frequency (Hz):"; ModulatingSignals "Internal generation of modulating signal(s)"; m "Modulation Index:"; Freq "Output voltage frequency (Hz):"; Phase "Output voltage phase (degrees):"; Ts "Sample time:"
      mask help:
      | The Discrete 3-phase PWM Generator block generates pulses for carrier-based
      | Pulse Width Modulation (PWM) converters. The block can be used to fire the
      | forced-commuted devices (FETs, GTOs, or IGBTs) of 2-level or 3-level converters
      | using a single  bridge or two bridges connected in twin configuration. Vectorized
      | outputs P1 and P2 contain  either 6 pulses (2-level) or 12 pulses (3-level).
      |
      | Use output P1 when operating in single-bridge configuration. The modulating
      | signals can be applied at Input 1 (Uref) and the synchronization signal at input 2 (wt).
      | Look under the mask' of the block to get a description of the pulse pattern.
      mask init: same as 03_ee_c/Wind Turbine/Control/Discrete 3-phase PWM Generator
      mask Help: This block is part of a subset of blocks in the Extras library that does not have documentation associated with it, other than the block mask description.
      mask TypeOptions ModulatorType: 2-level | 3-level
      mask TypeOptions ModulatorMode: Synchronized | Un-synchronized
      mask Callback ModulatorMode: powericon('psbcallbacks',gcb,'Discrete 3-phase PWM Generator',2);
      mask Callback ModulatingSignals: powericon('psbcallbacks',gcb,'Discrete 3-phase PWM Generator',5);
  Grid-side converter Control system : Subsystem
  MPPT & Pitch Control : Subsystem
  Measurement and Transformation : Subsystem
  PMSG-side converter Control system : Subsystem
  Terminator1 : Terminator
  Terminator3 : Terminator
  Unit Delay{1..2,5..6} (4 alike) : UnitDelay  SampleTime=Ts  HasFrameUpgradeWarning=on
  Inverter_Pulses : Outport
  Pitch_angle : Outport  Port=2
  Rectifier_Pulses : Outport  Port=3
  m : Outport  Port=4
  wires:
  MPPT & Pitch Control/2(Pitch (deg)) -> Unit Delay1/1
  MPPT & Pitch Control/1(Isq_ref) -> Unit Delay2/1
  Unit Delay2/1 -> PMSG-side converter Control system/2(Iq_ref)
  Unit Delay1/1 -> Pitch_angle/1
  Discrete 3-phase PWM Generator/1(P1) -> Inverter_Pulses/1
  Discrete 3-phase PWM Generator/2(P2) -> Terminator3/1
  Grid-side converter Control system/1(Uctrl_inverter) -> Unit Delay6/1
  Unit Delay6/1 -> Discrete 3-phase PWM Generator/1(Uref)
  Vabc_grid/1 -> Measurement and Transformation/1(Vabc_grid)
  Iabc_grid_conv/1 -> Measurement and Transformation/2(Iabc_gc)
  Vabc_LL_stator/1 -> Measurement and Transformation/3(Vabc_LL_s)
  Iabc_stator/1 -> Measurement and Transformation/4(Iabc_s)
  Vdc/1 -> Measurement and Transformation/5(Vdc)
  Qref/1 -> Measurement and Transformation/6(Qref)
  angle_rotor/1 -> Measurement and Transformation/7(angle_rotor)
  wr/1 -> Measurement and Transformation/8(wr)
  Discrete 3-phase PWM Generator1/1(P1) -> Rectifier_Pulses/1
  Discrete 3-phase PWM Generator1/2(P2) -> Terminator1/1
  Unit Delay5/1 -> Discrete 3-phase PWM Generator1/1(Uref)
  PMSG-side converter Control system/1(Uctrl_inverter) -> Unit Delay5/1
  Measurement and Transformation/1(m) -> m/1, Grid-side converter Control system/1(m), MPPT & Pitch Control/1(m), PMSG-side converter Control system/1(Idq_s)

== system 03_ee_c/Wind Turbine/Drive Train ==
  note: Wind turbine drive train based on a 2-masse model
  note: Turbine
  note: Shaft
  T_wt (pu) : Inport
  Generator speed (pu) : Inport  Port=2
  1_2H_WT : Gain  Gain=1/(2*H_WT)  SaturateOnIntegerOverflow=on  OutDataTypeStr=Inherit: Same as input  ParamDataTypeStr=Inherit: Same as input
  Discrete-Time Integrator : DiscreteIntegrator  InitialCondition=w_wt0  SampleTime=Ts  ICPrevOutput=DiscIntNeverNeededParam  ICPrevScaledInput=DiscIntNeverNeededParam
  Discrete-Time Integrator1 : DiscreteIntegrator  InitialCondition=torque0/Ksh  SampleTime=Ts  ICPrevOutput=DiscIntNeverNeededParam  ICPrevScaledInput=DiscIntNeverNeededParam
  Mutual damping : Gain  Gain=D_mutual  SaturateOnIntegerOverflow=on  OutDataTypeStr=Inherit: Same as input  ParamDataTypeStr=Inherit: Same as input
  Stiffness : Gain  Gain=Ksh  SaturateOnIntegerOverflow=on  OutDataTypeStr=Inherit: Same as input  ParamDataTypeStr=Inherit: Same as input
  Sum : Sum  Inputs=+-  InputSameDT=on  SaturateOnIntegerOverflow=on  OutDataTypeStr=Inherit: Same as first input
  Sum1 : Sum  Inputs=+-  InputSameDT=on  SaturateOnIntegerOverflow=on  OutDataTypeStr=Inherit: Same as first input
  Sum2 : Sum  InputSameDT=on  SaturateOnIntegerOverflow=on  OutDataTypeStr=Inherit: Same as first input
  wbase : Gain  Gain=wbase  SaturateOnIntegerOverflow=on  OutDataTypeStr=Inherit: Same as input  ParamDataTypeStr=Inherit: Same as input
  W_wt (pu) : Outport
  T_shaft (pu) : Outport  Port=2
  wires:
  T_wt (pu)/1 -> Sum/1
  Sum2/1 -> T_shaft (pu)/1, Sum/2
  Mutual damping/1 -> Sum2/2
  Sum1/1 -> Mutual damping/1, wbase/1
  Generator speed (pu)/1 -> Sum1/2
  Discrete-Time Integrator/1 -> W_wt (pu)/1, Sum1/1
  1_2H_WT/1 -> Discrete-Time Integrator/1
  Sum/1 -> 1_2H_WT/1
  Stiffness/1 -> Sum2/1
  Discrete-Time Integrator1/1 -> Stiffness/1
  wbase/1 -> Discrete-Time Integrator1/1

== system 03_ee_c/Wind Turbine/Wind Turbine ==
  W_wt (pu) : Inport
  Pitch angle (deg) : Inport  Port=2
  Wind speed (m/s) : Inport  Port=3
  ->pu : Gain  Gain=1/Prated
  Avoid div. by zero : Saturate  UpperLimit=inf  LowerLimit=eps
  "Avoid div. by zero " : Saturate  UpperLimit=inf  LowerLimit=eps
  Fcn1 : Fcn  Expr=K1*u[2]/u[1]
  Fcn2 : Fcn  Expr=c1*(c6*u[1] + (-c4 - c3*(2.5 + u[2]) + c2*(1/(u[1] + c7*(2.5 + u[2])) -c8/(1 + (2.5 + u[2])^3)))/exp(c5*(1/(u[1] + c7*(2.5 + u[2])) - c8/(1 + (2.5 + u[2])^3))))
  "K2*Cp*wind^3 " : Fcn  Expr=K2*u[1]^3*u[2]
  Mux : Mux  Inputs=2
  Mux1 : Mux  Inputs=2
  Mux2 : Mux  Inputs=2
  Product2 : Product  Inputs=*/  InputSameDT=on  SaturateOnIntegerOverflow=on  OutDataTypeStr=Inherit: Same as first input
  Tt (pu) : Outport
  wires:
  ->pu/1 -> Product2/1  "power_pu"
  Product2/1 -> Tt (pu)/1
  Wind speed (m/s)/1 -> Avoid div. by zero/1
  Fcn1/1 -> Mux1/1  "lambda"
  Mux1/1 -> Fcn2/1
  Mux/1 -> Fcn1/1
  Fcn2/1 -> Mux2/2  "Cp"
  Mux2/1 -> "K2*Cp*wind^3 "/1
  Pitch angle (deg)/1 -> Mux1/2
  W_wt (pu)/1 -> "Avoid div. by zero "/1
  Avoid div. by zero/1 -> Mux2/1, Mux/1
  "Avoid div. by zero "/1 -> Mux/2, Product2/2
  "K2*Cp*wind^3 "/1 -> ->pu/1

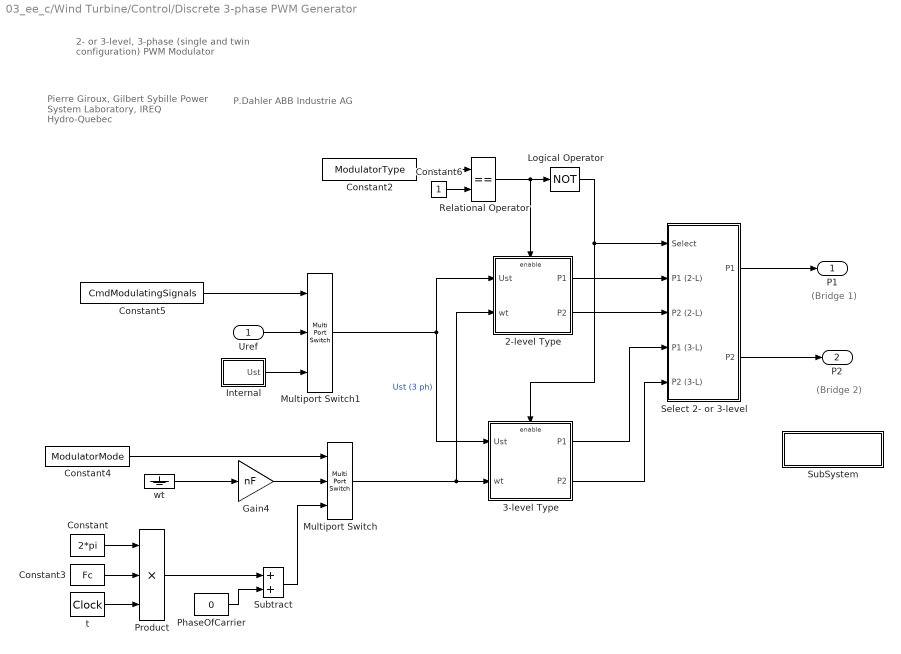
== system 03_ee_c/Wind Turbine/Control/Discrete 3-phase PWM Generator ==
  note: P.Dahler
      | ABB Industrie AG
  note: (Bridge 1)
  note: (Bridge 2)
  note: 2- or 3-level, 3-phase
      | (single and twin configuration)
      | PWM Modulator
  note: Pierre Giroux, Gilbert Sybille
      | Power System Laboratory, IREQ
      | Hydro-Quebec
  Uref : Inport
  2-level Type : Subsystem  TreatAsAtomicUnit=on
  3-level Type : Subsystem  TreatAsAtomicUnit=on
  Constant : Constant  Value=2*pi
  Constant2 : Constant  Value=ModulatorType
  Constant3 : Constant  Value=Fc
  Constant4 : Constant  Value=ModulatorMode
  Constant5 : Constant  Value=CmdModulatingSignals
  Constant6 : Constant
  Gain4 : Gain  Gain=nF  SaturateOnIntegerOverflow=on  OutDataTypeStr=Inherit: Same as input  ParamDataTypeStr=Inherit: Same as input
  Internal : Subsystem  mask(3-ph signal generator){m=m, Freq=Freq, Phase=Phase, Ts=Ts}
      mask prompts: m "Modulation Index:"; Freq "Output signal frequency (Hz):"; Phase "Output signal phase (degrees):"; Ts "Sample time:"
  Logical Operator : Logic  Operator=NOT
  Multiport Switch : MultiPortSwitch  Inputs=2  SaturateOnIntegerOverflow=off
  Multiport Switch1 : MultiPortSwitch  Inputs=2  SaturateOnIntegerOverflow=off
  PhaseOfCarrier : Constant  Value=0
  Product : Product  Inputs=3  InputSameDT=on  SaturateOnIntegerOverflow=on  OutDataTypeStr=Inherit: Same as first input
  Relational Operator : RelationalOperator  Operator===
  Select 2- or 3-level : Subsystem
  SubSystem : Subsystem
      mask Display: disp('Pulse pattern\ndescription')
  Subtract : Sum
  t : DigitalClock  SampleTime=Ts
  wt : Ground
  P1 : Outport
  P2 : Outport  Port=2
  wires:
  2-level Type/2(P2) -> Select 2- or 3-level/3(P2 (2-L))
  2-level Type/1(P1) -> Select 2- or 3-level/2(P1 (2-L))
  Select 2- or 3-level/1(P1) -> P1/1
  Select 2- or 3-level/2(P2) -> P2/1
  3-level Type/2(P2) -> Select 2- or 3-level/5(P2 (3-L))
  3-level Type/1(P1) -> Select 2- or 3-level/4(P1 (3-L))
  Logical Operator/1 -> Select 2- or 3-level/1(Select), 3-level Type/Enable
  Constant2/1 -> Relational Operator/1
  Relational Operator/1 -> Logical Operator/1, 2-level Type/Enable
  Constant6/1 -> Relational Operator/2
  Multiport Switch1/1 -> 3-level Type/1(Ust), 2-level Type/1(Ust)  "Ust (3 ph)"
  Multiport Switch/1 -> 3-level Type/2(wt), 2-level Type/2(wt)
  Constant/1 -> Product/1
  Constant3/1 -> Product/2
  t/1 -> Product/3
  wt/1 -> Gain4/1
  Constant4/1 -> Multiport Switch/1
  Gain4/1 -> Multiport Switch/2
  Internal/1("Ust ") -> Multiport Switch1/3
  Constant5/1 -> Multiport Switch1/1
  Uref/1 -> Multiport Switch1/2
  PhaseOfCarrier/1 -> Subtract/2
  Product/1 -> Subtract/1
  Subtract/1 -> Multiport Switch/3

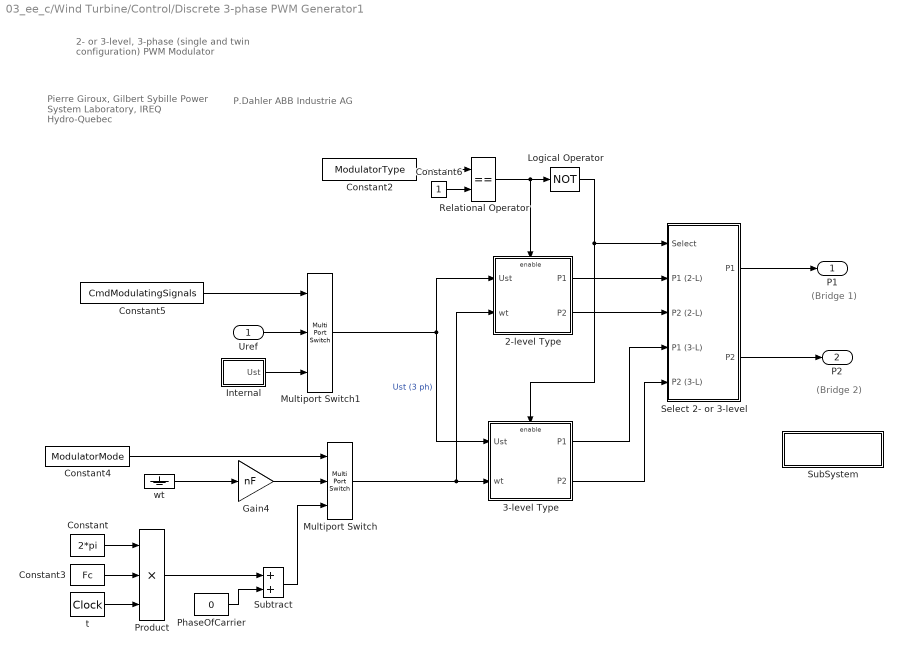
== system 03_ee_c/Wind Turbine/Control/Discrete 3-phase PWM Generator1 ==
  note: P.Dahler
      | ABB Industrie AG
  note: (Bridge 1)
  note: (Bridge 2)
  note: 2- or 3-level, 3-phase
      | (single and twin configuration)
      | PWM Modulator
  note: Pierre Giroux, Gilbert Sybille
      | Power System Laboratory, IREQ
      | Hydro-Quebec
  Uref : Inport
  2-level Type : Subsystem  TreatAsAtomicUnit=on
  3-level Type : Subsystem  TreatAsAtomicUnit=on
  Constant : Constant  Value=2*pi
  Constant2 : Constant  Value=ModulatorType
  Constant3 : Constant  Value=Fc
  Constant4 : Constant  Value=ModulatorMode
  Constant5 : Constant  Value=CmdModulatingSignals
  Constant6 : Constant
  Gain4 : Gain  Gain=nF  SaturateOnIntegerOverflow=on  OutDataTypeStr=Inherit: Same as input  ParamDataTypeStr=Inherit: Same as input
  Internal : Subsystem  mask(3-ph signal generator){m=m, Freq=Freq, Phase=Phase, Ts=Ts}
      mask prompts: m "Modulation Index:"; Freq "Output signal frequency (Hz):"; Phase "Output signal phase (degrees):"; Ts "Sample time:"
  Logical Operator : Logic  Operator=NOT
  Multiport Switch : MultiPortSwitch  Inputs=2  SaturateOnIntegerOverflow=off
  Multiport Switch1 : MultiPortSwitch  Inputs=2  SaturateOnIntegerOverflow=off
  PhaseOfCarrier : Constant  Value=0
  Product : Product  Inputs=3  InputSameDT=on  SaturateOnIntegerOverflow=on  OutDataTypeStr=Inherit: Same as first input
  Relational Operator : RelationalOperator  Operator===
  Select 2- or 3-level : Subsystem
  SubSystem : Subsystem
      mask Display: disp('Pulse pattern\ndescription')
  Subtract : Sum
  t : DigitalClock  SampleTime=Ts
  wt : Ground
  P1 : Outport
  P2 : Outport  Port=2
  wires:
  2-level Type/2(P2) -> Select 2- or 3-level/3(P2 (2-L))
  2-level Type/1(P1) -> Select 2- or 3-level/2(P1 (2-L))
  Select 2- or 3-level/1(P1) -> P1/1
  Select 2- or 3-level/2(P2) -> P2/1
  3-level Type/2(P2) -> Select 2- or 3-level/5(P2 (3-L))
  3-level Type/1(P1) -> Select 2- or 3-level/4(P1 (3-L))
  Logical Operator/1 -> Select 2- or 3-level/1(Select), 3-level Type/Enable
  Constant2/1 -> Relational Operator/1
  Relational Operator/1 -> Logical Operator/1, 2-level Type/Enable
  Constant6/1 -> Relational Operator/2
  Multiport Switch1/1 -> 3-level Type/1(Ust), 2-level Type/1(Ust)  "Ust (3 ph)"
  Multiport Switch/1 -> 3-level Type/2(wt), 2-level Type/2(wt)
  Constant/1 -> Product/1
  Constant3/1 -> Product/2
  t/1 -> Product/3
  wt/1 -> Gain4/1
  Constant4/1 -> Multiport Switch/1
  Gain4/1 -> Multiport Switch/2
  Internal/1("Ust ") -> Multiport Switch1/3
  Constant5/1 -> Multiport Switch1/1
  Uref/1 -> Multiport Switch1/2
  PhaseOfCarrier/1 -> Subtract/2
  Product/1 -> Subtract/1
  Subtract/1 -> Multiport Switch/3
